simulink model "NLADRC1"  (R2023a)
settings: Solver=VariableStepAuto  StartTime=0.0  StopTime=20  FixedStep=0.01  RelTol=1e-3
settings Model: Creator=belov  LastModifiedBy=belov

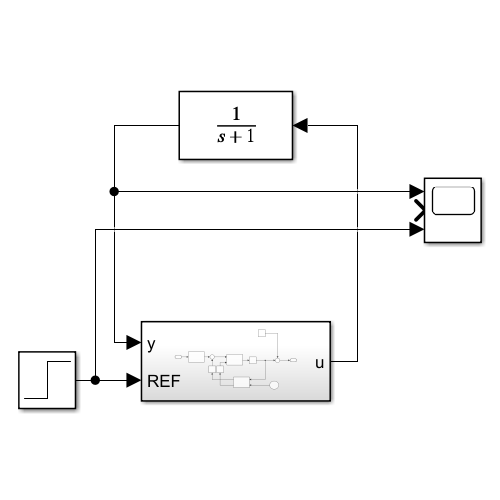
[thumbnail: Simulink's stored preview of the top-level diagram]
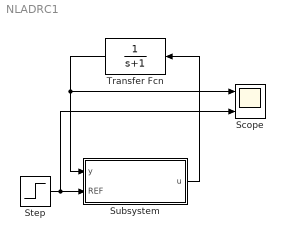
== system NLADRC1 ==
  Scope : Scope  NumInputPorts=3
  Step : Step  After=4  SampleTime=0.001
  Subsystem : Subsystem
  Transfer Fcn : TransferFcn  Denominator=[1 1]
  wires:
  Transfer Fcn/1 -> Subsystem/1(y), Scope/1
  Subsystem/1(u) -> Transfer Fcn/1
  Step/1 -> Subsystem/2(REF), Scope/3

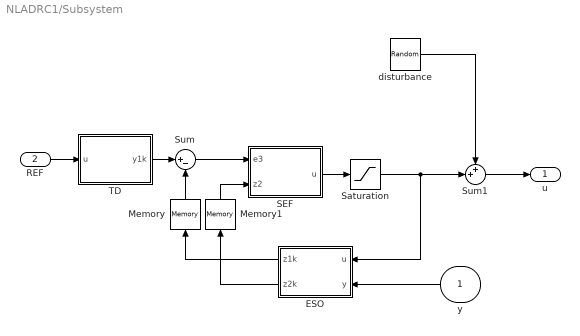
== system NLADRC1/Subsystem ==
  y : Inport
  REF : Inport  Port=2
  ESO : MATLAB Function  TreatAsAtomicUnit=on  SystemSampleTime=0.001
  Memory : Memory
  Memory1 : Memory
  SEF : MATLAB Function  TreatAsAtomicUnit=on  SystemSampleTime=0.001
  Saturation : Saturate  UpperLimit=10  LowerLimit=-10
  Sum : Sum  Inputs=|+-
  Sum1 : Sum  Inputs=++|
  TD : MATLAB Function  TreatAsAtomicUnit=on  SystemSampleTime=0.001
  disturbance : UniformRandomNumber  Minimum=-0.1  Maximum=0.1  SampleTime=0.1
  u : Outport
  wires:
  REF/1 -> TD/1(u)
  TD/1(y1k) -> Sum/1
  Sum/1 -> SEF/1(e3)
  ESO/1(z1k) -> Memory/1
  ESO/2(z2k) -> Memory1/1
  y/1 -> ESO/2(y)
  SEF/1(u) -> Saturation/1
  Memory/1 -> Sum/2
  Memory1/1 -> SEF/2(z2)
  Saturation/1 -> Sum1/2, ESO/1(u)
  disturbance/1 -> Sum1/1
  Sum1/1 -> u/1

== matlab function NLADRC1/Subsystem/TD ==
  data: u input; y1k output
function y1k = TD(u)
persistent y1k_1;

h = 0.001; %% 步长
delta1 = 0.01;
alpha1 = 1;
r = 10; %% 用于调整趋于平稳的速度

if isempty(y1k_1)
    y1k_1 = 0;
end

e1 = y1k_1 - u;

%%%% fal计算
e1abs = abs(e1);
fal = 0;
if e1abs <= delta1
    fal = e1abs ^ alpha1 * sign(e1);
else 
    fal = e1 / (delta1 ^ (1 - alpha1));
end

y1k = y1k_1 - r * h * fal;

y1k_1 = y1k;

end

== matlab function NLADRC1/Subsystem/SEF ==
  data: e3 input; u output; z2 input
function u = SEF(e3, z2)

alpha3 = 1;
delta3 = 0.01;
%%%% fal
e3abs = abs(e3);
fal = 0;
if e3abs <= delta3
    fal = e3abs ^ alpha3 * sign(e3);
else 
    fal = e3 / (delta3 ^ (1 - alpha3));
end

kp = 10; % 需要调整
u0 = kp * fal;
b0 = 1;
u = (u0 - z2) / b0;

end

== matlab function NLADRC1/Subsystem/ESO ==
  data: u input; z1k output; y input; z2k output
function [z1k, z2k]= ESO(u, y)
persistent z1k_1 z2k_1;
if isempty(z1k_1)
    z1k_1 = 0;
end
if isempty(z2k_1)
    z2k_1 = 0;
end
h = 0.001; %% 步长，需要注意所有模块的步长都相同
e2 = z1k_1 - y;

alpha2 = 1;
delta2 = 0.01;

wc = 5; % 这个也需要调节
wo = wc * 3;

beta21 = 2 * wo;
beta22 = wo ^ 2;

b0 = 1; % 这个需要调节的参数，好像需要和其它函数里对应

%%%% fal计算
e2abs = abs(e2);
fal = 0;
if e2abs <= delta2
    fal = e2abs ^ alpha2 * sign(e2);
else 
    fal = e2 / (delta2 ^ (1 - alpha2));
end

z1k = h * (z2k_1 - beta21 * fal + b0 * u) + z1k_1;
z2k = z2k_1 - h * beta22 * fal;

z1k_1 = z1k;
z2k_1 = z2k;

end
